simulink model "NNPID"  (R2024b)
settings: Solver=FixedStepDiscrete  StartTime=0.0  StopTime=10.0  FixedStep=0.001  RelTol=1e-3
settings Model: Creator=Sapna Kotecha  LastModifiedBy=Sapna Kotecha

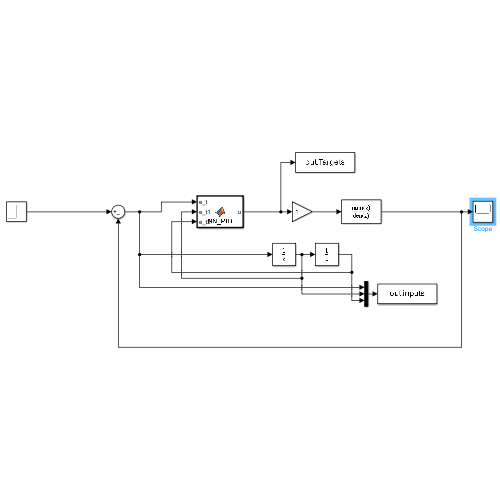
[thumbnail: Simulink's stored preview of the top-level diagram]
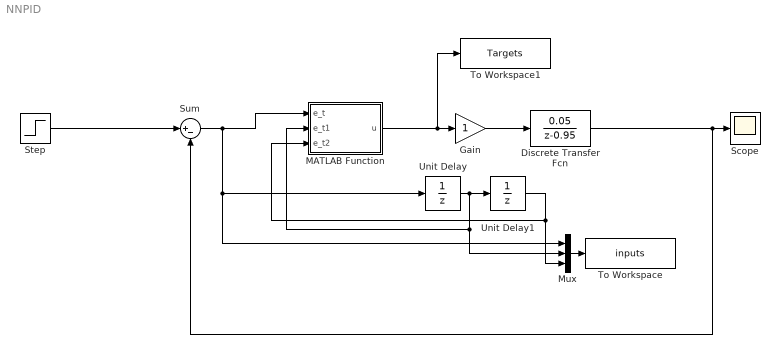
== system NNPID ==
  Discrete Transfer Fcn : DiscreteTransferFcn  Numerator=[0.05]  Denominator=[1 -0.95]
  Gain : Gain
  MATLAB Function : MATLAB Function  TreatAsAtomicUnit=on
  Mux : Mux  Inputs=3
  Scope : Scope
  Step : Step  Time=0  SampleTime=0
  Sum : Sum  Inputs=|+-
  To Workspace : ToWorkspace  VariableName=inputs  SampleTime=-1
      settings: MaxDataPoints=99999
  To Workspace1 : ToWorkspace  VariableName=Targets  SampleTime=-1
      settings: MaxDataPoints=99999
  Unit Delay : UnitDelay  SampleTime=-1  HasFrameUpgradeWarning=on
  Unit Delay1 : UnitDelay  SampleTime=-1  HasFrameUpgradeWarning=on
  wires:
  Step/1 -> Sum/1
  MATLAB Function/1(u) -> To Workspace1/1, Gain/1
  Gain/1 -> Discrete Transfer Fcn/1
  Discrete Transfer Fcn/1 -> Sum/2, Scope/1
  Unit Delay/1 -> MATLAB Function/2(e_t1), Mux/2, Unit Delay1/1
  Unit Delay1/1 -> Mux/3, MATLAB Function/3(e_t2)
  Mux/1 -> To Workspace/1
  Sum/1 -> Unit Delay/1, Mux/1, MATLAB Function/1(e_t)

== matlab function NNPID/MATLAB Function ==
  data: e_t input; u output; e_t1 input; e_t2 input
function u = NN_PID(e_t, e_t1, e_t2)
%#codegen
% Neural Network-based PID Emulator
% Inputs:  e_t, e_t1, e_t2  → current and past error values (scalars)
% Output:  u                → control signal (scalar)

% === Neural Network Weights ===

% Layer 1: 10 neurons, input size = 3
W1 = [ ...
     0.0402  -0.1475   0.0544;
     0.2482   0.3096  -0.2572;
    -0.2259   0.0725   0.0717;
     0.0095  -0.0498   0.1815;
     0.0950   0.4045   0.3226;
    -0.1308  -0.0205   0.1035;
    -0.1072  -0.0972   0.0803;
    -0.0275   0.3782   0.2684;
     0.4062   0.3912   0.1264;
     0.3457   0.5745   0.2248 ];

b1 = [ ...
     0.0323;
    -0.0131;
     0.0000;
     0.0819;
    -0.0336;
     0.0000;
     0.2132;
    -0.0199;
    -0.2041;
    -0.0478 ];

% Layer 2: 5 neurons, input size = 10
W2 = [ ...
     0.1103   0.1258  -0.0102  -0.0599  -0.2899   0.1533  -0.0830  -0.1884  -0.2296  -0.3475;
    -0.1008   0.0187  -0.0241  -0.0530  -0.1193  -0.0770   0.0198  -0.2721  -0.0319  -0.2713;
    -0.1070  -0.0754   0.0319   0.0624  -0.1222   0.0371   0.0547  -0.0746  -0.0193   0.0480;
    -0.0540   0.0489   0.0313  -0.0062  -0.4096  -0.0226   0.1420  -0.3968  -0.2239  -0.3518;
    -0.3013  -0.3666  -0.0865   0.1622  -0.1504   0.1117   0.2924   0.1133  -0.3832  -0.3493 ];

b2 = [ ...
     0.4037;
     0.2739;
    -0.0004;
     0.4839;
     0.7343 ];

% Output layer: 1 neuron, input size = 5
W3 = [0.6635  0.4344  0.0212  0.8354  -0.9815];
b3 =  0.9486;

% === Forward Pass ===
x = [e_t; e_t1; e_t2];           % Input vector

% Layer 1 → ReLU
z1 = W1 * x + b1;
a1 = max(0, z1);

% Layer 2 → ReLU
z2 = W2 * a1 + b2;
a2 = max(0, z2);

% Output layer → Linear
u = W3 * a2 + b3;

% Optional: saturate output between 0 and 1
% u = min(max(u, 0), 1);
end
